simulink model "actuator_dynamics_kalman"  (R2019a)
settings: Solver=VariableStepAuto  StartTime=0.0  StopTime=100  RelTol=1e-3
InitFcn:
  | initialize_lab_c_kalman
values from neighbouring files (symbols this model uses):
  A = [0, 	0	,  1.1320	, 	0		, -1.0000 ... (first row only)    [initialize_lab_c.m]    (also in initialize_lab_c_kalman.m; no_disturbances.mat = [0 0 0 0 0 0 -0.0538 0 0.0485 -0.2909 1.132 -0.1712 ... (25 )
  B = [	0		, 0		, 	0 ... (first row only)    [initialize_lab_c.m]    (also in initialize_lab_c_kalman.m; no_disturbances.mat = [0 -0.12 0 4.419 1.575 0 1 0 0 0 0 0 ... (15 elements, 5x3)])
  C = [  1, 0, 0, 0, 0 ... (first row only)    [initialize_lab_c.m]    (also in initialize_lab_c_kalman.m; no_disturbances.mat = [1 0 0 0 1 0 0 0 1 0 0 0 ... (15 elements, 3x5)])
  D = zeros(3)    [initialize_lab_c.m]    (also in initialize_lab_c_kalman.m; no_disturbances.mat = [0  0  0; 0  0  0; 0  0  0])
  Kf = [0.910312414486 -0.0156881663418 0.323774090813 0.0384957916935 -0.0222349654056 -0.0156881663418 0.341721504352 -0.0124401259868 0.0454656343337 -0.046565981811 0.323774090813 -0.0124401259868 ... (15 elements, 5x3)]    [no_disturbances.mat]
  L = lqr(A-Kf*C,B,Q,R)    [initialize_lab_c_kalman.m]    (also in no_disturbances.mat = [-62.1347904879 0.684280536131 -78.3504918375 -0.28851971530)
  Lr = pinv(M*inv(B*L-A)*B)    [initialize_lab_c_kalman.m]    (also in no_disturbances.mat = [-62.1347904879  -0.076288731515  56.111048242; 0.6842805361)
libraries: cstblocks x3
settings Model: Creator=marbla-6  LastModifiedBy=Martin

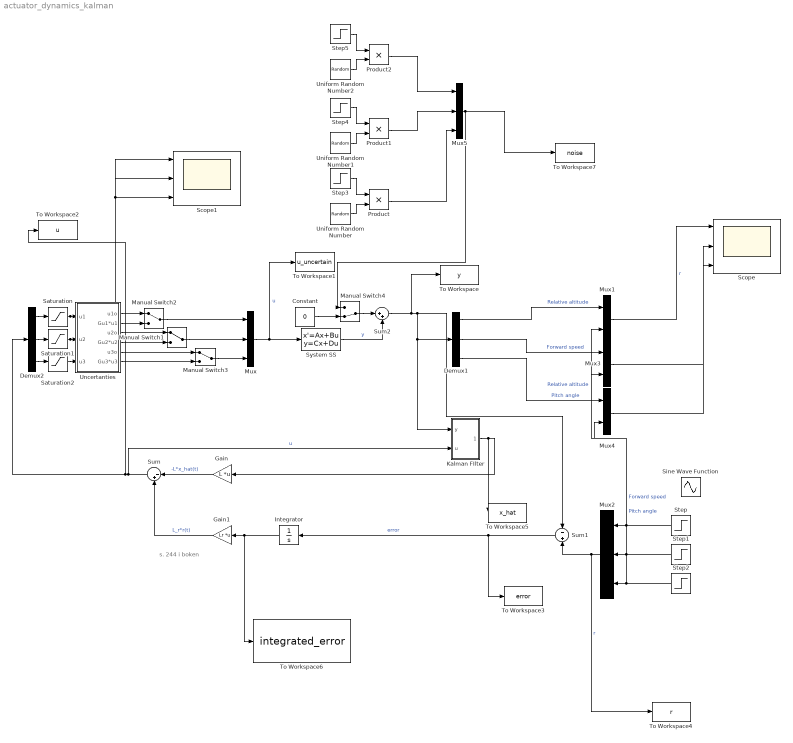
== system actuator_dynamics_kalman ==
  note: s. 244 i boken
  Constant : Constant  Value=0
  Demux1 : Demux  Outputs=3
  Demux2 : Demux  Outputs=3
  Gain : Gain  Gain=L  Multiplication=Matrix(K*u)
  Gain1 : Gain  Gain=Lr  Multiplication=Matrix(K*u)
  Integrator : Integrator
  Kalman FIlter : Subsystem
  Manual Switch1 : ManualSwitch
  Manual Switch2 : ManualSwitch
  Manual Switch3 : ManualSwitch
  Manual Switch4 : ManualSwitch  CurrentSetting=0
  Mux : Mux  Inputs=3
  Mux1 : Mux  Inputs=2
  Mux2 : Mux  Inputs=3
  Mux3 : Mux  Inputs=2
  Mux4 : Mux  Inputs=2
  Mux5 : Mux  Inputs=3
  Product : Product
  Product1 : Product
  Product2 : Product
  Saturation : Saturate  UpperLimit=900  LowerLimit=-900
  Saturation1 : Saturate  UpperLimit=20  LowerLimit=-20
  Saturation2 : Saturate  UpperLimit=90  LowerLimit=-90
  Scope : Scope  NumInputPorts=3
  Scope1 : Scope  NumInputPorts=3
  Sine Wave Function : Sin  Amplitude=50  Bias=500  Frequency=.5  SampleTime=0
  Step : Step  Time=20  After=20  SampleTime=0
  Step1 : Step  Time=50  After=20  SampleTime=0
  Step2 : Step  Time=70  After=3  SampleTime=0
  Step3 : Step  Time=0  Before=1  SampleTime=0
  Step4 : Step  Time=0  Before=1  SampleTime=0
  Step5 : Step  Time=0  Before=1  SampleTime=0
  Sum : Sum  Inputs=|-+
  Sum1 : Sum  Inputs=-+
  Sum2 : Sum  Inputs=|++
  System SS : StateSpace  A=A  B=B  C=C  D=D  InitialCondition=0
  To Workspace : ToWorkspace  VariableName=y  SaveFormat=Timeseries  SampleTime=-1
  To Workspace1 : ToWorkspace  VariableName=u_uncertain  SaveFormat=Timeseries  SampleTime=-1
  To Workspace2 : ToWorkspace  VariableName=u  SaveFormat=Timeseries  SampleTime=-1
  To Workspace3 : ToWorkspace  VariableName=error  SaveFormat=Timeseries  SampleTime=-1
  To Workspace4 : ToWorkspace  VariableName=r  SaveFormat=Timeseries  SampleTime=-1
  To Workspace5 : ToWorkspace  VariableName=x_hat  SaveFormat=Timeseries  SampleTime=-1
  To Workspace6 : ToWorkspace  VariableName=integrated_error  SaveFormat=Timeseries  SampleTime=-1
  To Workspace7 : ToWorkspace  VariableName=noise  SaveFormat=Timeseries  SampleTime=-1
  Uncertanties : Subsystem
  Uniform Random Number : UniformRandomNumber  Minimum=-.1  Maximum=.1  SampleTime=0.1
  Uniform Random Number1 : UniformRandomNumber  SampleTime=0.1
  Uniform Random Number2 : UniformRandomNumber  SampleTime=0.1
  wires:
  Manual Switch3/1 -> Mux/3
  Manual Switch1/1 -> Mux/2
  Uncertanties/4(Gu2*u2) -> Manual Switch1/2
  Manual Switch2/1 -> Mux/1
  Uncertanties/2(Gu1*u1) -> Manual Switch2/2
  Uncertanties/6(Gu3*u3) -> Manual Switch3/2
  Uncertanties/3(u2o) -> Manual Switch1/1
  Uncertanties/5(u3o) -> Manual Switch3/1
  Uncertanties/1(u1o) -> Manual Switch2/1
  Gain/1 -> Sum/1  "-L*x_hat(t)"
  Gain1/1 -> Sum/2  "L_r*r(t)"
  Demux1/1 -> Mux1/1  "Relative altitude"
  Mux1/1 -> Scope/1  "r"
  Constant/1 -> Manual Switch4/2
  Demux1/2 -> Mux3/1  "Forward speed"
  Demux1/3 -> Mux4/1  "Pitch angle"
  Demux2/1 -> Saturation/1
  Demux2/2 -> Saturation1/1
  Demux2/3 -> Saturation2/1
  Integrator/1 -> Gain1/1, To Workspace6/1
  Kalman FIlter/1(x_hat) -> Gain/1, To Workspace5/1
  Manual Switch4/1 -> Sum2/1
  Mux2/1 -> Sum1/2, To Workspace4/1  "r"
  Mux3/1 -> Scope/2
  Mux4/1 -> Scope/3
  Mux5/1 -> To Workspace7/1, Manual Switch4/1
  Mux/1 -> System SS/1, To Workspace1/1  "u"
  Product1/1 -> Mux5/2
  Product2/1 -> Mux5/1
  Product/1 -> Mux5/3
  Saturation1/1 -> Scope1/2, Scope1/3, Uncertanties/2(u2)
  Saturation2/1 -> Uncertanties/3(u3)
  Saturation/1 -> Uncertanties/1(u1), Scope1/1
  Step1/1 -> Mux2/2, Mux3/2  "Forward speed"
  Step2/1 -> Mux2/3, Mux4/2  "Pitch angle"
  Step3/1 -> Product/1
  Step4/1 -> Product1/1
  Step5/1 -> Product2/1
  Step/1 -> Mux2/1, Mux1/2  "Relative altitude"
  Sum1/1 -> Integrator/1, To Workspace3/1  "error"
  Sum2/1 -> Kalman FIlter/1(y), Demux1/1, Sum1/1, To Workspace/1
  Sum/1 -> Demux2/1, To Workspace2/1, Kalman FIlter/2(u)  "u"
  System SS/1 -> Sum2/2  "y"
  Uniform Random Number1/1 -> Product1/2
  Uniform Random Number2/1 -> Product2/2
  Uniform Random Number/1 -> Product/2

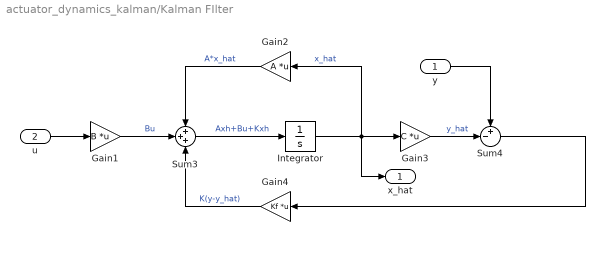
== system actuator_dynamics_kalman/Kalman FIlter ==
  y : Inport
  u : Inport  Port=2
  Gain1 : Gain  Gain=B  Multiplication=Matrix(K*u)
  Gain2 : Gain  Gain=A  Multiplication=Matrix(K*u)
  Gain3 : Gain  Gain=C  Multiplication=Matrix(K*u)
  Gain4 : Gain  Gain=Kf  Multiplication=Matrix(K*u)
  Integrator : Integrator
  Sum3 : Sum  Inputs=+++
  Sum4 : Sum  Inputs=+-|
  x_hat : Outport
  wires:
  Gain4/1 -> Sum3/3  "K(y-y_hat)"
  Gain3/1 -> Sum4/2  "y_hat"
  Gain1/1 -> Sum3/2  "Bu"
  Integrator/1 -> x_hat/1, Gain3/1, Gain2/1  "x_hat"
  Sum3/1 -> Integrator/1  "Axh+Bu+Kxh"
  Gain2/1 -> Sum3/1  "A*x_hat"
  Sum4/1 -> Gain4/1
  u/1 -> Gain1/1
  y/1 -> Sum4/1

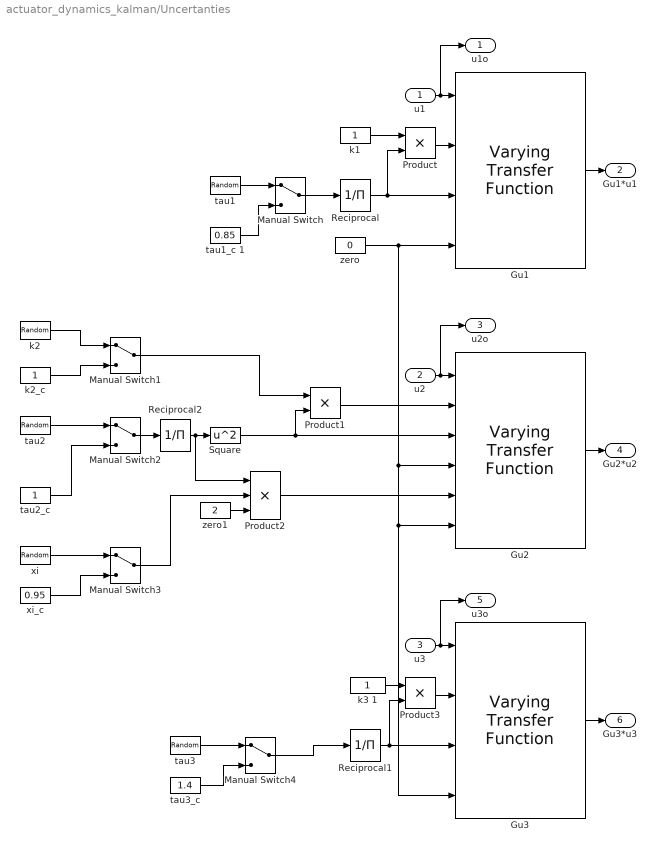
== system actuator_dynamics_kalman/Uncertanties ==
  u1 : Inport
  u2 : Inport  Port=2
  u3 : Inport  Port=3
  Gu1 : cstblocks/Linear Parameter Varying/Varying Transfer Function  N=1
      settings: SourceProductName=Control System Toolbox
  Gu2 : cstblocks/Linear Parameter Varying/Varying Transfer Function  N=2
      settings: SourceProductName=Control System Toolbox
  Gu3 : cstblocks/Linear Parameter Varying/Varying Transfer Function  N=1
      settings: SourceProductName=Control System Toolbox
  Manual Switch{,1..4} (5 alike) : ManualSwitch
  Product : Product
  Product1 : Product
  Product2 : Product  Inputs=3
  Product3 : Product
  Reciprocal : Product  Inputs=/
  Reciprocal1 : Product  Inputs=/
  Reciprocal2 : Product  Inputs=/
  Square : Math  Operator=square  SaturateOnIntegerOverflow=on
  "k1 " : Constant
  k2 : UniformRandomNumber  Minimum=0.9+1e-6  Maximum=1.1-1e-6  SampleTime=0.1
  k2_c : Constant
  k3 1 : Constant
  tau1 : UniformRandomNumber  Minimum=0.5+1e-6  Maximum=1.2-1e-6  SampleTime=0.1
  tau1_c 1 : Constant  Value=0.85
  tau2 : UniformRandomNumber  Minimum=0.5+1e-6  Maximum=2.5-1e-6  SampleTime=0.1
  tau2_c : Constant
  tau3 : UniformRandomNumber  Minimum=1+1e-6  Maximum=1.8-1e-6  SampleTime=0.1
  tau3_c : Constant  Value=1.4
  xi : UniformRandomNumber  Minimum=0.9+1e-6  Maximum=1-1e-6  SampleTime=0.1
  xi_c : Constant  Value=0.95
  zero : Constant  Value=0
  zero1 : Constant  Value=2
  u1o : Outport
  Gu1*u1 : Outport  Port=2
  u2o : Outport  Port=3
  Gu2*u2 : Outport  Port=4
  u3o : Outport  Port=5
  Gu3*u3 : Outport  Port=6
  wires:
  Gu2/1 -> Gu2*u2/1
  Manual Switch3/1 -> Product2/2
  tau3_c/1 -> Manual Switch4/2
  u1/1 -> u1o/1, Gu1/1
  Reciprocal/1 -> Gu1/3, Product/2
  Gu3/1 -> Gu3*u3/1
  Reciprocal1/1 -> Gu3/3, Product3/2
  Product1/1 -> Gu2/2
  Square/1 -> Gu2/3, Product1/2
  k2/1 -> Manual Switch1/1
  k3 1/1 -> Product3/1
  xi_c/1 -> Manual Switch3/2
  zero1/1 -> Product2/3
  Manual Switch/1 -> Reciprocal/1
  Manual Switch4/1 -> Reciprocal1/1
  Reciprocal2/1 -> Product2/1, Square/1
  xi/1 -> Manual Switch3/1
  zero/1 -> Gu1/4, Gu3/4, Gu2/6, Gu2/4
  tau2_c/1 -> Manual Switch2/2
  Product3/1 -> Gu3/2
  "k1 "/1 -> Product/1
  Manual Switch2/1 -> Reciprocal2/1
  u2/1 -> u2o/1, Gu2/1
  Product/1 -> Gu1/2
  Product2/1 -> Gu2/5
  k2_c/1 -> Manual Switch1/2
  tau1/1 -> Manual Switch/1
  Manual Switch1/1 -> Product1/1
  tau3/1 -> Manual Switch4/1
  u3/1 -> u3o/1, Gu3/1
  tau1_c 1/1 -> Manual Switch/2
  tau2/1 -> Manual Switch2/1
  Gu1/1 -> Gu1*u1/1
